simulink model "Projekt_ABS_Sim_4_2"  (R2024b)
settings: Solver=VariableStepAuto  StartTime=0.0  StopTime=10  RelTol=1e-3
values from neighbouring files (symbols this model uses):
  c1 = 0.857    [Projekt_ABS.m]
  c11 = 1.2801    [Projekt_ABS.m]
  c2 = 33.822    [Projekt_ABS.m]
  c22 = 23.99    [Projekt_ABS.m]
  c3 = 0.347    [Projekt_ABS.m]
  c33 = 0.52    [Projekt_ABS.m]
  c4 = 0.035    [Projekt_ABS.m]
  c44 = 0.03    [Projekt_ABS.m]
  g = 9.81    [Projekt_ABS.m]
  J = 1.6    [Projekt_ABS.m]
  m = 1200    [Projekt_ABS.m]
  Mb = 900    [Projekt_ABS.m]
  R = 0.315    [Projekt_ABS.m]
  Ts = 0.01    [Projekt_ABS.m]
  V0 = 40    [Projekt_ABS.m]
undefined symbols (not defined in the file or in its folder): DiscIntNeverNeededParam
libraries: simulink x4, slpidlib x2
settings Model: Creator=abc  LastModifiedBy=abc

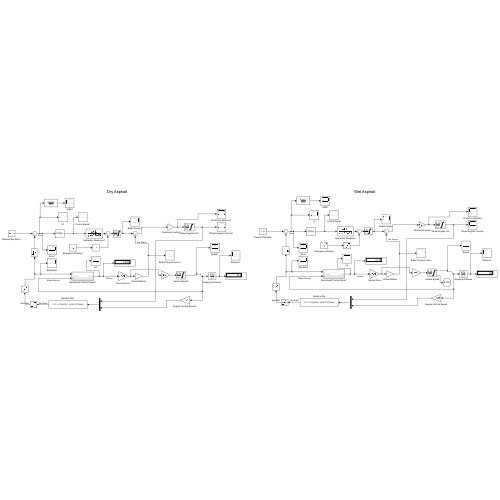
[thumbnail: Simulink's stored preview of the top-level diagram]
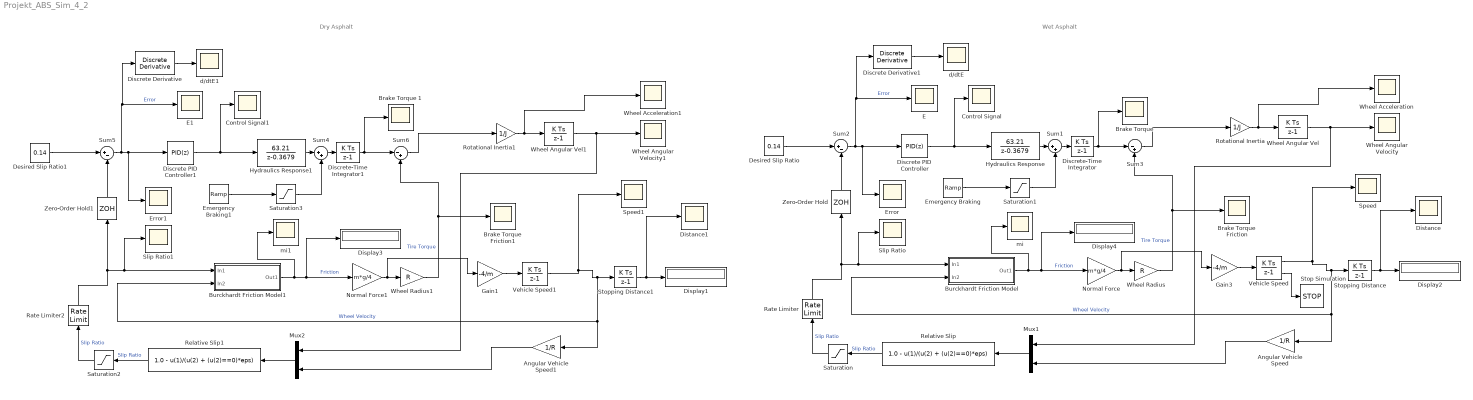
== system Projekt_ABS_Sim_4_2 ==
  note: Wet Asphalt
  note: Dry Asphalt
  Angular Vehicle Speed : Gain  Gain=1/R
  Angular Vehicle Speed1 : Gain  Gain=1/R
  "Brake Torque " : Scope
  Brake Torque 1 : Scope
  Brake Torque Friction : Scope
  Brake Torque Friction1 : Scope
  Burckhardt Friction Model : Subsystem
  Burckhardt Friction Model1 : Subsystem
  Control Signal : Scope
  Control Signal1 : Scope
  Desired Slip Ratio : Constant  Value=0.14  SampleTime=0.01
  Desired Slip Ratio1 : Constant  Value=0.14  SampleTime=0.01
  Discrete Derivative : simulink/Discrete/Discrete Derivative  gainval=1.0  ICPrevScaledInput=0.0  OutMin=[]  OutMax=[]  OutDataType=fixdt(1, 16)  OutScaling=2^-10  DoSatur=off
  Discrete Derivative1 : simulink/Discrete/Discrete Derivative  gainval=1.0  ICPrevScaledInput=0.0  OutMin=[]  OutMax=[]  OutDataType=fixdt(1, 16)  OutScaling=2^-10  DoSatur=off
  Discrete PID Controller : slpidlib/PID Controller  Controller=PID  Form=Parallel  TimeDomain=Discrete-time  UseExternalTs=off  SampleTime=0.01  IntegratorMethod=Forward Euler  FilterMethod=Forward Euler  ControllerParametersSource=internal  P=175  I=10  UseKiTs=off  D=27  UseExternalDerivativeSource=off  N=150  UseFilter=on  TunerSelectOption=Transfer Function Based (PID Tuner App)  InitialConditionSource=internal  InitialConditionForIntegrator=0  InitialConditionForFilter=0  DifferentiatorICPrevScaledInput=0  ExternalReset=none  TrackingMode=off  Kt=1  LimitOutput=off  SatLimitsSource=internal  UpperSaturationLimit=inf  LowerSaturationLimit=-inf  LinearizeAsGain=off  AntiWindupMode=none  Kb=1  LimitIntegrator=off  UpperIntegratorSaturationLimit=inf  LowerIntegratorSaturationLimit=-inf  POutMin=[]  POutMax=[]  IOutMin=[]  IOutMax=[]  DOutMin=[]  DOutMax=[]  NOutMin=[]  NOutMax=[]  SumOutMin=[]  SumOutMax=[]  SaturationOutMin=[]  SaturationOutMax=[]  PParamMin=[]  PParamMax=[]  IParamMin=[]  IParamMax=[]  DParamMin=[]  DParamMax=[]  NParamMin=[]  NParamMax=[]  KbParamMin=[]  KbParamMax=[]  KtParamMin=[]  KtParamMax=[]  KbOutMin=[]  KbOutMax=[]  KtOutMin=[]  KtOutMax=[]  IntegratorOutMin=[]  IntegratorOutMax=[]  FilterOutMin=[]  FilterOutMax=[]  SumI1OutMin=[]  SumI1OutMax=[]  SumI2OutMin=[]  SumI2OutMax=[]  SumI3OutMin=[]  SumI3OutMax=[]  SumI4OutMin=[]  SumI4OutMax=[]  SumDOutMin=[]  SumDOutMax=[]  DifferentiatorOutMin=[]  DifferentiatorOutMax=[]  FilterDiffOutCoefMin=[]  FilterDiffOutCoefMax=[]  ReciprocalOutMin=[]  ReciprocalOutMax=[]  SumDenOutMin=[]  SumDenOutMax=[]  SumNumOutMin=[]  SumNumOutMax=[]  DivideOutMin=[]  DivideOutMax=[]  UdiffTsProdOutMin=[]  UdiffTsProdOutMax=[]  NTsProdOutMin=[]  NTsProdOutMax=[]  UintegralTsProdOutMin=[]  UintegralTsProdOutMax=[]  UngainTsProdOutMin=[]  UngainTsProdOutMax=[]  ClampingZeroOutDataTypeStr=Inherit: Inherit via back propagation  ClampingZeroOutMin=[]  ClampingZeroOutMax=[]  FilterDenConstantOutDataTypeStr=Inherit: Inherit via back propagation  FilterDenConstantOutMin=[]  FilterDenConstantOutMax=[]  PCopyOutDataTypeStr=Inherit: Inherit via back propagation  PCopyOutMin=[]  PCopyOutMax=[]  NCopyOutDataTypeStr=Inherit: Inherit via back propagation  NCopyOutMin=[]  NCopyOutMax=[]  IntegratorContinuousStateAttributes=''  IntegratorStateMustResolveToSignalObject=off  IntegratorRTWStateStorageClass=Auto  FilterContinuousStateAttributes=''  FilterStateMustResolveToSignalObject=off  FilterRTWStateStorageClass=Auto  ParallelPVariant=InternalParameters  IdealPVariant=Disabled  IVariant=InternalParameters  DVariant=InternalParameters  IntegratorVariant=Discrete  SatVariant=Disabled  AWVariant=Passthrough  PCopyVariant=Disabled  TRVariant=Disabled  FdbkBlocksVariant=Forward  IdealPFdbkVariant=Disabled  SatFdbkVariant=Disabled  DerivativeFilterVariant=ForwardEulerFilter  NVariant=InternalParameters  NCopyVariant=Disabled  FilterICVariant=InternalICsFilter  IntegratorICVariant=InternalICs  ExternalResetVariant=Disabled  TRSumVariant=Passthrough  SumFdbkVariant=Disabled  SumVariant=Sum_PID  TsampFilterVariant=InternalTs  TsampNgainVariant=Passthrough  TsampIntegralVariant=Disabled_SignalSpec  ExternalSaturationOutDataTypeStr=Inherit: Same as second input  DerivativeSourceVariant=ErrorSignal  PreIntVariant=InternalPreInt
      settings: LibrarySourceBlock=simulink/Discrete/Discrete PID Controller
  Discrete PID Controller1 : slpidlib/PID Controller  Controller=PID  Form=Parallel  TimeDomain=Discrete-time  UseExternalTs=off  SampleTime=0.01  IntegratorMethod=Forward Euler  FilterMethod=Forward Euler  ControllerParametersSource=internal  P=175  I=10  UseKiTs=off  D=27  UseExternalDerivativeSource=off  N=150  UseFilter=on  TunerSelectOption=Transfer Function Based (PID Tuner App)  InitialConditionSource=internal  InitialConditionForIntegrator=0  InitialConditionForFilter=0  DifferentiatorICPrevScaledInput=0  ExternalReset=none  TrackingMode=off  Kt=1  LimitOutput=off  SatLimitsSource=internal  UpperSaturationLimit=inf  LowerSaturationLimit=-inf  LinearizeAsGain=off  AntiWindupMode=none  Kb=1  LimitIntegrator=off  UpperIntegratorSaturationLimit=inf  LowerIntegratorSaturationLimit=-inf  POutMin=[]  POutMax=[]  IOutMin=[]  IOutMax=[]  DOutMin=[]  DOutMax=[]  NOutMin=[]  NOutMax=[]  SumOutMin=[]  SumOutMax=[]  SaturationOutMin=[]  SaturationOutMax=[]  PParamMin=[]  PParamMax=[]  IParamMin=[]  IParamMax=[]  DParamMin=[]  DParamMax=[]  NParamMin=[]  NParamMax=[]  KbParamMin=[]  KbParamMax=[]  KtParamMin=[]  KtParamMax=[]  KbOutMin=[]  KbOutMax=[]  KtOutMin=[]  KtOutMax=[]  IntegratorOutMin=[]  IntegratorOutMax=[]  FilterOutMin=[]  FilterOutMax=[]  SumI1OutMin=[]  SumI1OutMax=[]  SumI2OutMin=[]  SumI2OutMax=[]  SumI3OutMin=[]  SumI3OutMax=[]  SumI4OutMin=[]  SumI4OutMax=[]  SumDOutMin=[]  SumDOutMax=[]  DifferentiatorOutMin=[]  DifferentiatorOutMax=[]  FilterDiffOutCoefMin=[]  FilterDiffOutCoefMax=[]  ReciprocalOutMin=[]  ReciprocalOutMax=[]  SumDenOutMin=[]  SumDenOutMax=[]  SumNumOutMin=[]  SumNumOutMax=[]  DivideOutMin=[]  DivideOutMax=[]  UdiffTsProdOutMin=[]  UdiffTsProdOutMax=[]  NTsProdOutMin=[]  NTsProdOutMax=[]  UintegralTsProdOutMin=[]  UintegralTsProdOutMax=[]  UngainTsProdOutMin=[]  UngainTsProdOutMax=[]  ClampingZeroOutDataTypeStr=Inherit: Inherit via back propagation  ClampingZeroOutMin=[]  ClampingZeroOutMax=[]  FilterDenConstantOutDataTypeStr=Inherit: Inherit via back propagation  FilterDenConstantOutMin=[]  FilterDenConstantOutMax=[]  PCopyOutDataTypeStr=Inherit: Inherit via back propagation  PCopyOutMin=[]  PCopyOutMax=[]  NCopyOutDataTypeStr=Inherit: Inherit via back propagation  NCopyOutMin=[]  NCopyOutMax=[]  IntegratorContinuousStateAttributes=''  IntegratorStateMustResolveToSignalObject=off  IntegratorRTWStateStorageClass=Auto  FilterContinuousStateAttributes=''  FilterStateMustResolveToSignalObject=off  FilterRTWStateStorageClass=Auto  ParallelPVariant=InternalParameters  IdealPVariant=Disabled  IVariant=InternalParameters  DVariant=InternalParameters  IntegratorVariant=Discrete  SatVariant=Disabled  AWVariant=Passthrough  PCopyVariant=Disabled  TRVariant=Disabled  FdbkBlocksVariant=Forward  IdealPFdbkVariant=Disabled  SatFdbkVariant=Disabled  DerivativeFilterVariant=ForwardEulerFilter  NVariant=InternalParameters  NCopyVariant=Disabled  FilterICVariant=InternalICsFilter  IntegratorICVariant=InternalICs  ExternalResetVariant=Disabled  TRSumVariant=Passthrough  SumFdbkVariant=Disabled  SumVariant=Sum_PID  TsampFilterVariant=InternalTs  TsampNgainVariant=Passthrough  TsampIntegralVariant=Disabled_SignalSpec  ExternalSaturationOutDataTypeStr=Inherit: Same as second input  DerivativeSourceVariant=ErrorSignal  PreIntVariant=InternalPreInt
      settings: LibrarySourceBlock=simulink/Discrete/Discrete PID Controller
  Discrete-Time Integrator : DiscreteIntegrator  SampleTime=0.01  LimitOutput=on  UpperSaturationLimit=Mb  LowerSaturationLimit=0  ICPrevOutput=DiscIntNeverNeededParam  ICPrevScaledInput=DiscIntNeverNeededParam
  Discrete-Time Integrator1 : DiscreteIntegrator  SampleTime=0.01  LimitOutput=on  UpperSaturationLimit=Mb  LowerSaturationLimit=0  ICPrevOutput=DiscIntNeverNeededParam  ICPrevScaledInput=DiscIntNeverNeededParam
  Display{1..4} (4 alike) : Display
  Distance : Scope
  Distance1 : Scope
  E : Scope
  E1 : Scope
  Emergency Braking : simulink/Sources/Ramp  slope=Mb*2  start=0  InitialOutput=0
  Emergency Braking1 : simulink/Sources/Ramp  slope=Mb*2  start=0  InitialOutput=0
  Error : Scope
  Error1 : Scope
  Gain1 : Gain  Gain=-4/m
  Gain3 : Gain  Gain=-4/m
  Hydraulics Response : DiscreteTransferFcn  Numerator=[63.21]  Denominator=[1 -0.3679]  SampleTime=Ts
  Hydraulics Response1 : DiscreteTransferFcn  Numerator=[63.21]  Denominator=[1 -0.3679]  SampleTime=Ts
  Mux1 : Mux  Inputs=2
  Mux2 : Mux  Inputs=2
  Normal Force : Gain  Gain=m*g/4
  Normal Force1 : Gain  Gain=m*g/4
  Rate Limiter : RateLimiter  RisingSlewLimit=1.5  FallingSlewLimit=-1.5  SampleTimeMode=inherited
  Rate Limiter2 : RateLimiter  RisingSlewLimit=1.5  FallingSlewLimit=-1.5  SampleTimeMode=inherited
  Relative Slip : Fcn  Expr=1.0 - u(1)/(u(2) + (u(2)==0)*eps)
  Relative Slip1 : Fcn  Expr=1.0 - u(1)/(u(2) + (u(2)==0)*eps)
  Rotational Inertia : Gain  Gain=1/J
  Rotational Inertia1 : Gain  Gain=1/J
  Saturation : Saturate  UpperLimit=1  LowerLimit=0
  Saturation1 : Saturate  UpperLimit=Mb  LowerLimit=0
  Saturation2 : Saturate  UpperLimit=1  LowerLimit=0
  Saturation3 : Saturate  UpperLimit=Mb  LowerLimit=0
  Slip Ratio : Scope
  Slip Ratio1 : Scope
  Speed : Scope
  Speed1 : Scope
  Stop Simulation : Stop
  Stopping Distance : DiscreteIntegrator  SampleTime=0.01  ICPrevOutput=DiscIntNeverNeededParam  ICPrevScaledInput=DiscIntNeverNeededParam
  Stopping Distance1 : DiscreteIntegrator  SampleTime=0.01  ICPrevOutput=DiscIntNeverNeededParam  ICPrevScaledInput=DiscIntNeverNeededParam
  Sum1 : Sum  Inputs=|++
  Sum2 : Sum  Inputs=|+-
  Sum3 : Sum  Inputs=|-+
  Sum4 : Sum  Inputs=|++
  Sum5 : Sum  Inputs=|+-
  Sum6 : Sum  Inputs=|-+
  Vehicle Speed : DiscreteIntegrator  InitialCondition=V0  SampleTime=0.01  LimitOutput=on  UpperSaturationLimit=1000  LowerSaturationLimit=0  ShowSaturationPort=on  ICPrevOutput=DiscIntNeverNeededParam  ICPrevScaledInput=DiscIntNeverNeededParam
  Vehicle Speed1 : DiscreteIntegrator  InitialCondition=V0  SampleTime=0.01  LimitOutput=on  UpperSaturationLimit=1000  LowerSaturationLimit=0  ICPrevOutput=DiscIntNeverNeededParam  ICPrevScaledInput=DiscIntNeverNeededParam
  Wheel Acceleration : Scope
  Wheel Acceleration1 : Scope
  Wheel Angular Vel : DiscreteIntegrator  InitialCondition=V0/R  SampleTime=0.01  LimitOutput=on  UpperSaturationLimit=1000  LowerSaturationLimit=0  ICPrevOutput=DiscIntNeverNeededParam  ICPrevScaledInput=DiscIntNeverNeededParam
  Wheel Angular Vel1 : DiscreteIntegrator  InitialCondition=V0/R  SampleTime=0.01  LimitOutput=on  UpperSaturationLimit=1000  LowerSaturationLimit=0  ICPrevOutput=DiscIntNeverNeededParam  ICPrevScaledInput=DiscIntNeverNeededParam
  Wheel Angular Velocity : Scope
  Wheel Angular Velocity1 : Scope
  Wheel Radius : Gain  Gain=R
  Wheel Radius1 : Gain  Gain=R
  Zero-Order Hold : ZeroOrderHold  SampleTime=0.01
  Zero-Order Hold1 : ZeroOrderHold  SampleTime=0.01
  d/dtE : Scope
  d/dtE1 : Scope
  mi : Scope
  mi1 : Scope
  wires:
  Sum3/1 -> Rotational Inertia/1
  Vehicle Speed/1 -> Stopping Distance/1, Burckhardt Friction Model/2(In2), Angular Vehicle Speed/1, Speed/1  "Wheel Velocity"
  Stopping Distance/1 -> Distance/1, Display2/1
  Wheel Angular Vel/1 -> Wheel Angular Velocity/1, Mux1/1
  Relative Slip/1 -> Saturation/1  "Slip Ratio"
  Burckhardt Friction Model/1(Out1) -> mi/1, Display4/1, Normal Force/1  "Friction"
  Mux1/1 -> Relative Slip/1
  Normal Force/1 -> Gain3/1, Wheel Radius/1
  Rotational Inertia/1 -> Wheel Angular Vel/1, Wheel Acceleration/1
  Wheel Radius/1 -> Brake Torque Friction/1, Sum3/2  "Tire Torque"
  Angular Vehicle Speed/1 -> Mux1/2
  Zero-Order Hold/1 -> Sum2/2
  Gain3/1 -> Vehicle Speed/1
  Rate Limiter/1 -> Zero-Order Hold/1, Slip Ratio/1, Burckhardt Friction Model/1(In1)
  Saturation/1 -> Rate Limiter/1  "Slip Ratio"
  Sum2/1 -> Discrete PID Controller/1, Error/1, Discrete Derivative1/1, E/1  "Error"
  Desired Slip Ratio/1 -> Sum2/1
  Discrete-Time Integrator/1 -> "Brake Torque "/1, Sum3/1
  Vehicle Speed/2 -> Stop Simulation/1
  Discrete PID Controller/1 -> Control Signal/1, Hydraulics Response/1
  Hydraulics Response/1 -> Sum1/1
  Sum1/1 -> Discrete-Time Integrator/1
  Emergency Braking/1 -> Saturation1/1
  Saturation1/1 -> Sum1/2
  Saturation3/1 -> Sum4/2
  Discrete PID Controller1/1 -> Control Signal1/1, Hydraulics Response1/1
  Sum4/1 -> Discrete-Time Integrator1/1
  Wheel Angular Vel1/1 -> Wheel Angular Velocity1/1, Mux2/1
  Desired Slip Ratio1/1 -> Sum5/1
  Burckhardt Friction Model1/1(Out1) -> mi1/1, Display3/1, Normal Force1/1  "Friction"
  Gain1/1 -> Vehicle Speed1/1
  Mux2/1 -> Relative Slip1/1
  Sum6/1 -> Rotational Inertia1/1
  Normal Force1/1 -> Gain1/1, Wheel Radius1/1
  Discrete-Time Integrator1/1 -> Brake Torque 1/1, Sum6/1
  Wheel Radius1/1 -> Brake Torque Friction1/1, Sum6/2  "Tire Torque"
  Saturation2/1 -> Rate Limiter2/1  "Slip Ratio"
  Hydraulics Response1/1 -> Sum4/1
  Zero-Order Hold1/1 -> Sum5/2
  Relative Slip1/1 -> Saturation2/1  "Slip Ratio"
  Stopping Distance1/1 -> Distance1/1, Display1/1
  Rotational Inertia1/1 -> Wheel Angular Vel1/1, Wheel Acceleration1/1
  Emergency Braking1/1 -> Saturation3/1
  Vehicle Speed1/1 -> Speed1/1, Stopping Distance1/1, Burckhardt Friction Model1/2(In2), Angular Vehicle Speed1/1  "Wheel Velocity"
  Angular Vehicle Speed1/1 -> Mux2/2
  Rate Limiter2/1 -> Zero-Order Hold1/1, Slip Ratio1/1, Burckhardt Friction Model1/1(In1)
  Sum5/1 -> Discrete PID Controller1/1, Error1/1, Discrete Derivative/1, E1/1  "Error"
  Discrete Derivative/1 -> d/dtE1/1
  Discrete Derivative1/1 -> d/dtE/1

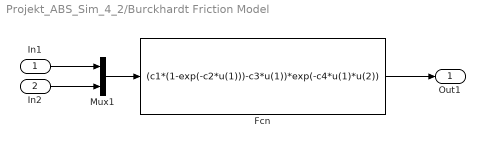
== system Projekt_ABS_Sim_4_2/Burckhardt Friction Model ==
  In1 : Inport
  In2 : Inport  Port=2
  Fcn : Fcn  Expr=(c1*(1-exp(-c2*u(1)))-c3*u(1))*exp(-c4*u(1)*u(2))
  Mux1 : Mux  Inputs=2
  Out1 : Outport
  wires:
  In2/1 -> Mux1/2
  Mux1/1 -> Fcn/1
  In1/1 -> Mux1/1
  Fcn/1 -> Out1/1

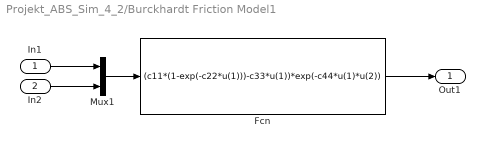
== system Projekt_ABS_Sim_4_2/Burckhardt Friction Model1 ==
  In1 : Inport
  In2 : Inport  Port=2
  Fcn : Fcn  Expr=(c11*(1-exp(-c22*u(1)))-c33*u(1))*exp(-c44*u(1)*u(2))
  Mux1 : Mux  Inputs=2
  Out1 : Outport
  wires:
  In2/1 -> Mux1/2
  Mux1/1 -> Fcn/1
  In1/1 -> Mux1/1
  Fcn/1 -> Out1/1
